simulink model "lab1B"  (R2018b)
settings: Solver=VariableStepAuto  StartTime=0.0  StopTime=10.0  MaxStep=1e-4  RelTol=1e-3
libraries: simulink x1
settings Model: Creator=joshua  LastModifiedBy=joshua

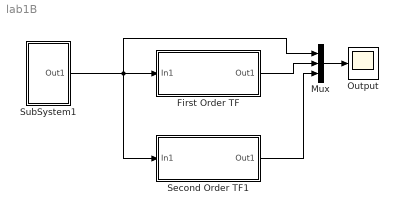
== system lab1B ==
  First Order TF : Subsystem  mask{a=1}
      mask prompts: a "param"
  Mux : Mux  Inputs=3
  Output : Scope
  Second Order TF1 : Subsystem  mask{a=1}
      mask prompts: a "param"
  SubSystem1 : Subsystem  mask{f=1}
      mask prompts: f "function"
  wires:
  SubSystem1/1(Out1) -> First Order TF/1(In1), Mux/1, Second Order TF1/1(In1)
  First Order TF/1(Out1) -> Mux/2
  Mux/1 -> Output/1
  Second Order TF1/1(Out1) -> Mux/3

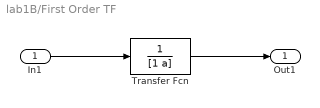
== system lab1B/First Order TF ==
  In1 : Inport
  Transfer Fcn : TransferFcn  Denominator=[1 a]
  Out1 : Outport
  wires:
  In1/1 -> Transfer Fcn/1
  Transfer Fcn/1 -> Out1/1

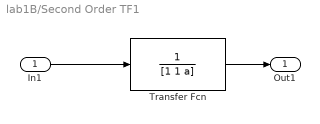
== system lab1B/Second Order TF1 ==
  In1 : Inport
  Transfer Fcn : TransferFcn  Denominator=[1 1 a]
  Out1 : Outport
  wires:
  Transfer Fcn/1 -> Out1/1
  In1/1 -> Transfer Fcn/1

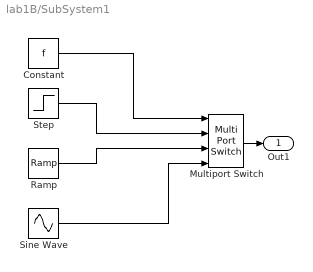
== system lab1B/SubSystem1 ==
  Constant : Constant  Value=f
  Multiport Switch : MultiPortSwitch
  Ramp : simulink/Sources/Ramp  slope=1  start=0  InitialOutput=0
  Sine Wave : Sin  Frequency=2*pi  SampleTime=0
  Step : Step  Time=0.5  SampleTime=0
  Out1 : Outport
  wires:
  Constant/1 -> Multiport Switch/1
  Step/1 -> Multiport Switch/2
  Multiport Switch/1 -> Out1/1
  Ramp/1 -> Multiport Switch/3
  Sine Wave/1 -> Multiport Switch/4
